simulink model "PMSM_gm_can_outside_Trq_attack"  (R2023a)
settings: Solver=VariableStepAuto  StartTime=0  StopTime=t_sim  RelTol=1e-3
values from neighbouring files (symbols this model uses):
  chosen_cycle = input('Enter the number of the desired driver cycle-choose: \n 1 for Artemis Motorway Driving cycle \n 2 for WHVC \n 3 for ECE urban driving cycle \n 4 for cruise control \n')    [pmsm_g.m]
  J = 0.03    [pmsm_g.m]
  Rated_Cap = 145.5    [pmsm_g.m]
  SOC0 = 1    [pmsm_g.m]
  T_peak = 450    [pmsm_g.m]
  Tire_rad = 0.33435    [pmsm_g.m]
undefined symbols (not defined in the file or in its folder): canChannel, DiscIntNeverNeededParam, sigbuilder_block
libraries: fl_lib x26, nesl_utility x13, sdl_lib x10, canlib x9, canmsglib x8, autolibshared x4, batteryecm_lib x2, ee_lib x2, simulink x1, SignalEditorBlockLib x1
(part 1 of 2)
settings Model: Creator=SMISTOKI  LastModifiedBy=Sadek
settings DebuggingCC: AlgebraicLoopMsg=none

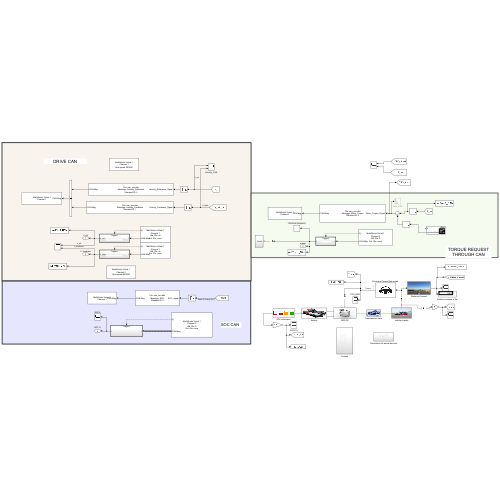
[thumbnail: Simulink's stored preview of the top-level diagram]
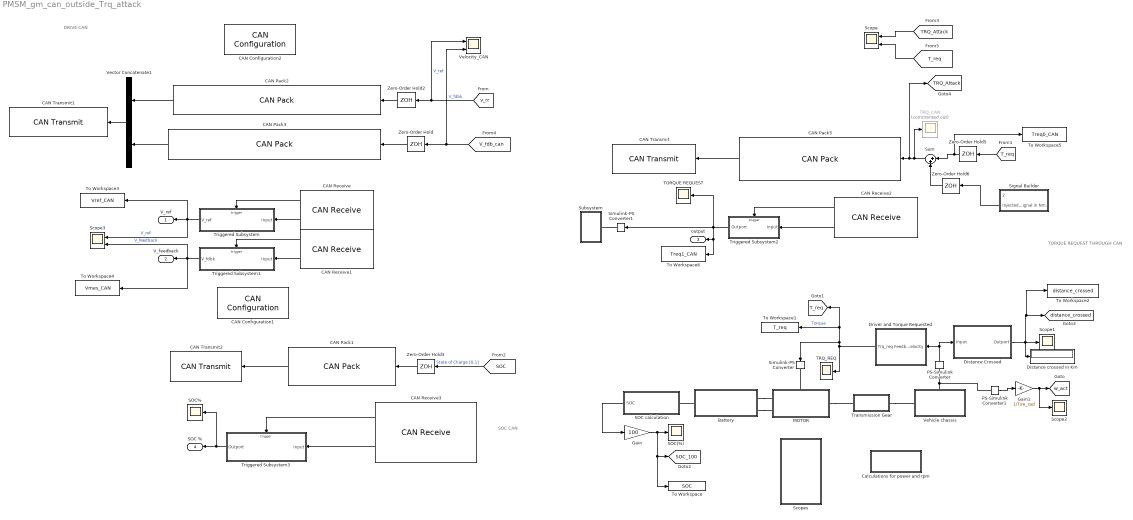
== system PMSM_gm_can_outside_Trq_attack ==
  note: SOC CAN
  note: TORQUE REQUEST THROUGH CAN
  note: DRIVE CAN
  Battery : Subsystem
      settings: PortSchema="{\"entries\":[{\"content\":{\"sides\":[{\"content\":{},\"type\":\"ConnectorPlacement.EquallySpacedRectSide\",\"uuid\":\"d6ab2843-64d8-482c-9d15-215691b6cf54\"},{\"content\":{\"side\":\"RIGHT\"},\"type\":\"ConnectorPlacement.EquallySpacedRectSide\",\"uuid\":\"de85a474-0fdd-49ed-84f8-84d3f4b19d16\"},{\"content\":{\"connectorIds\":[\"LConn1\",\"LConn2\"],\"side\":\"TOP\"},\"type\":\"ConnectorPlacement.EquallySpacedRectSide\",\"uuid\":\"2ee0526d-0566-4e29-bcb7-1bed3def4007\"},{\"content\":{\"connectorIds\":[\"RConn1\"],\"side\":\"BOTTOM\"},\"type\":\"ConnectorPlacement.EquallySpacedRectSide\",\"uuid\":\"606897e6-0cfb-4cd6-a0a0-49c9c925cf1d\"}]},\"type\":\"ConnectorPlacement.EquallySpacedConnector\",\"uuid\":\"bf6b65d6-9bac-4f3f-a275-26fa16d307ff\"}],\"packageUris\":[\"http://schema.mathworks.com/mf0/Connector/R2020b\"],\"version\":\"1.0\"}"
      mask Display: image('$imagefile'); % Use "Edit Image" on toolstrip to change.
  CAN Configuration1 : canlib/CAN Configuration  BlockHandle=30.0001  Device=MathWorks Virtual 1 (Channel 2)  DeviceMenu=MathWorks Virtual 1 (Channel 2)  ObjConstructor=canChannel('MathWorks', 'Virtual 1', 2)  BusSpeed=500000  EnableBitParameters=off  AckMode=Normal
  CAN Configuration2 : canlib/CAN Configuration  BlockHandle=31.0001  Device=MathWorks Virtual 1 (Channel 1)  DeviceMenu=MathWorks Virtual 1 (Channel 1)  ObjConstructor=canChannel('MathWorks', 'Virtual 1', 1)  BusSpeed=500000  EnableBitParameters=off  AckMode=Normal
  CAN Pack1 : canmsglib/CAN Pack  CANdbFile=C:\Users\Sadek\OneDrive - Politecnico di Torino\Final model\can_ecu.dbc  MsgList=SOC  MsgName=SOC  MsgIDType=Standard (11-bit identifier)  MsgIdentifier=5  MsgLength=8  Remote=off  ApplyMinMax=off  BusOutput=off  SignalInfo={'SOC_signal','0','64','LE','double','Standard','0','1','-20','0','100'}
      settings: LibrarySourceBlock=canlib/CAN Pack  DataFormat=CANdb specified signals
  CAN Pack2 : canmsglib/CAN Pack  CANdbFile=C:\Users\Sadek\OneDrive - Politecnico di Torino\Final model\can_ecu.dbc  MsgList=Velocity_Reference  MsgName=Velocity_Reference  MsgIDType=Standard (11-bit identifier)  MsgIdentifier=2  MsgLength=8  Remote=off  ApplyMinMax=off  BusOutput=off  SignalInfo={'Velocity_Reference_Signal','0','64','LE','double','Standard','0','1','-20','0','10000'}
      settings: LibrarySourceBlock=canlib/CAN Pack  DataFormat=CANdb specified signals
  CAN Pack3 : canmsglib/CAN Pack  CANdbFile=C:\Users\Sadek\OneDrive - Politecnico di Torino\Final model\can_ecu.dbc  MsgList=Velocity_Feedback  MsgName=Velocity_Feedback  MsgIDType=Standard (11-bit identifier)  MsgIdentifier=1  MsgLength=8  Remote=off  ApplyMinMax=off  BusOutput=off  SignalInfo={'Velocity_Feedback_Signal','0','64','LE','double','Standard','0','1','-20','0','10000'}
      settings: LibrarySourceBlock=canlib/CAN Pack  DataFormat=CANdb specified signals
  CAN Pack5 : canmsglib/CAN Pack  CANdbFile=C:\Users\Sadek\OneDrive - Politecnico di Torino\Final model\can_ecu.dbc  MsgList=Motor_Torque  MsgName=Motor_Torque  MsgIDType=Standard (11-bit identifier)  MsgIdentifier=0  MsgLength=8  Remote=off  ApplyMinMax=off  BusOutput=off  SignalInfo={'Motor_Torque_Signal','0','64','LE','signed','Standard','0','1','-20','-50000','50000'}
      settings: LibrarySourceBlock=canlib/CAN Pack  DataFormat=CANdb specified signals
  CAN Receive : canlib/CAN Receive  BlockHandle=44.0001  Device=MathWorks Virtual 1 (Channel 1)  DeviceMenu=MathWorks Virtual 1 (Channel 1)  ObjConstructor=canChannel('MathWorks', 'Virtual 1', 1)  EnableStandardIDsFilter=off  StdIDsCombo=Allow all  StandardIDs=0  EnableExtendedIDsFilter=off  ExtIDsCombo=Block all  ExtendedIDs=0  SampleTime=0.01  MsgsPerTimestep=all  InternalFilterUpdateStatus=on  BusOutput=off
  CAN Receive1 : canlib/CAN Receive  BlockHandle=47.0001  Device=MathWorks Virtual 1 (Channel 1)  DeviceMenu=MathWorks Virtual 1 (Channel 1)  ObjConstructor=canChannel('MathWorks', 'Virtual 1', 1)  EnableStandardIDsFilter=off  StdIDsCombo=Allow all  StandardIDs=0  EnableExtendedIDsFilter=off  ExtIDsCombo=Block all  ExtendedIDs=0  SampleTime=0.01  MsgsPerTimestep=all  InternalFilterUpdateStatus=on  BusOutput=off
  CAN Receive2 : canlib/CAN Receive  BlockHandle=50.0001  Device=MathWorks Virtual 1 (Channel 2)  DeviceMenu=MathWorks Virtual 1 (Channel 2)  ObjConstructor=canChannel('MathWorks', 'Virtual 1', 2)  EnableStandardIDsFilter=off  StdIDsCombo=Allow only  StandardIDs=0  EnableExtendedIDsFilter=off  ExtIDsCombo=Block all  ExtendedIDs=0  SampleTime=0.01  MsgsPerTimestep=all  InternalFilterUpdateStatus=on  BusOutput=off
  CAN Receive3 : canlib/CAN Receive  BlockHandle=53.0001  Device=MathWorks Virtual 1 (Channel 2)  DeviceMenu=MathWorks Virtual 1 (Channel 2)  ObjConstructor=canChannel('MathWorks', 'Virtual 1', 2)  EnableStandardIDsFilter=off  StdIDsCombo=Allow only  StandardIDs=5  EnableExtendedIDsFilter=off  ExtIDsCombo=Block all  ExtendedIDs=0  SampleTime=0.01  MsgsPerTimestep=all  InternalFilterUpdateStatus=on  BusOutput=on
  CAN Transmit : canlib/CAN Transmit  BlockHandle=56.0001  Device=MathWorks Virtual 1 (Channel 1)  DeviceMenu=MathWorks Virtual 1 (Channel 1)  ObjConstructor=canChannel('MathWorks', 'Virtual 1', 1)  EnableEventTransmit=off  EnablePeriodicTransmit=off  MessagePeriod=1.000
  CAN Transmit1 : canlib/CAN Transmit  BlockHandle=58.0001  Device=MathWorks Virtual 1 (Channel 1)  DeviceMenu=MathWorks Virtual 1 (Channel 1)  ObjConstructor=canChannel('MathWorks', 'Virtual 1', 1)  EnableEventTransmit=off  EnablePeriodicTransmit=off  MessagePeriod=1.000
  CAN Transmit2 : canlib/CAN Transmit  BlockHandle=60.0001  Device=MathWorks Virtual 1 (Channel 1)  DeviceMenu=MathWorks Virtual 1 (Channel 1)  ObjConstructor=canChannel('MathWorks', 'Virtual 1', 1)  EnableEventTransmit=off  EnablePeriodicTransmit=off  MessagePeriod=1.000
  Calculations for power and rpm : Subsystem
  Distance Crossed : Subsystem
      mask Display: image('$imagefile'); % Use "Edit Image" on toolstrip to change.
  Distance crossed in Km : Display
  "Driver and Torque Requested " : Subsystem
      mask Display: image('$imagefile'); % Use "Edit Image" on toolstrip to change.
  Gain : Gain  Gain=100
  Gain1 : Gain  Gain=1/Tire_rad
  MOTOR : Subsystem
      settings: PortSchema="{\"entries\":[{\"content\":{\"sides\":[{\"content\":{\"connectorIds\":[\"LConn1\",\"LConn2\"]},\"type\":\"ConnectorPlacement.EquallySpacedRectSide\",\"uuid\":\"2895f6cb-f09c-4811-a438-7c51f6a6223f\"},{\"content\":{\"connectorIds\":[\"RConn1\"],\"side\":\"RIGHT\"},\"type\":\"ConnectorPlacement.EquallySpacedRectSide\",\"uuid\":\"62dfe04d-e035-47c8-a996-d867f35d8ae8\"},{\"content\":{\"connectorIds\":[\"LConn3\"],\"side\":\"TOP\"},\"type\":\"ConnectorPlacement.EquallySpacedRectSide\",\"uuid\":\"0c3302b4-833a-415e-90fd-2f2c79a3935c\"}]},\"type\":\"ConnectorPlacement.EquallySpacedConnector\",\"uuid\":\"ac0404f8-73ea-47f6-91f8-dc1d39a3ba60\"}],\"packageUris\":[\"http://schema.mathworks.com/mf0/Connector/R2020b\"],\"version\":\"1.0\"}"
      mask Display: image('$imagefile'); % Use "Edit Image" on toolstrip to change.
  PS-Simulink Converter : nesl_utility/PS-Simulink Converter  PhysicalDomain=network_engine_domain  SubClassName=ps_output  LeftPortType=input  RightPortType=output  PseudoPeriodic=off  Frequencies=[]  VectorFormat=inherit  Unit=inherit  AffineConversion=off
  PS-Simulink Converter1 : nesl_utility/PS-Simulink Converter  PhysicalDomain=network_engine_domain  SubClassName=ps_output  LeftPortType=input  RightPortType=output  PseudoPeriodic=off  Frequencies=[]  VectorFormat=inherit  Unit=inherit  AffineConversion=off
  "SOC calculation " : Subsystem
      mask Display: image('$imagefile'); % Use "Edit Image" on toolstrip to change.
  SOC% : Scope
  SOC(%) : Scope
  Scope : Scope  NumInputPorts=2
  Scope1 : Scope
  Scope2 : Scope
  Scope3 : Scope  NumInputPorts=2
  Scopes : Subsystem
  Signal Builder : Subsystem  Tag=STV Subsys  LoadFcn=sigbuilder_block('load');  StartFcn=sigbuilder_block('start');  StopFcn=sigbuilder_block('stop');  ClipboardFcn=sigbuilder_block('clipboard');  mask(Sigbuilder block){tuvar=[0:10]}
      mask help: Simulink:masks:SigbuilderBlock_MD
      mask init:
      | if ~strcmp(get_param(bdroot(gcbh),'SimulationStatus'),'stopped') tuvar = sigbuilder_block('maskInit'); end
      settings: CopyFcn=sigbuilder_block('copy');  DeleteFcn=sigbuilder_block('delete');  ModelCloseFcn=sigbuilder_block('modelClose');  PreSaveFcn=sigbuilder_block('preSave');  PauseFcn=sigbuilder_block('pause');  ContinueFcn=sigbuilder_block('continue');  NameChangeFcn=sigbuilder_block('namechange');  OpenFcn=sigbuilder_block('open',[5.4 5.4 1141.2 580.8 ]);  CloseFcn=sigbuilder_block('close');
      mask Display: plot(0, 0, 100, 100,[2, 2, 32, 32, 2], [68, 8, 8, 68, 68],[32, 2], [38, 38], [32, 19, 2],[53, 60, 44], [32, 17, 17, 2],[16, 16, 31, 31]);txt = getActiveGroup(gcbh);text(2, 100, txt,'verticalAlignment', 'top');
  Simulink-PS Converter : nesl_utility/Simulink-PS Converter  PhysicalDomain=network_engine_domain  SubClassName=ps_input  LeftPortType=input  RightPortType=output  PseudoPeriodic=off  Frequencies=[]  NoiseDistribution=none  NoiseParameters=[]  Unit=1  AffineConversion=off  FilteringAndDerivatives=provide  SimscapeFilterOrder=1  InputFilterTimeConstant=0.001  UdotUserProvided=0
  Simulink-PS Converter1 : nesl_utility/Simulink-PS Converter  PhysicalDomain=network_engine_domain  SubClassName=ps_input  LeftPortType=input  RightPortType=output  PseudoPeriodic=off  Frequencies=[]  NoiseDistribution=none  NoiseParameters=[]  Unit=1  AffineConversion=off  FilteringAndDerivatives=provide  SimscapeFilterOrder=1  InputFilterTimeConstant=0.001  UdotUserProvided=0
  Subsystem : Subsystem
  Sum : Sum  Inputs=|++
  TORQUE REQUEST : Scope
  TRQ_CAN : Scope  Commented=on
  TRQ_REQ : Scope
  To Workspace : ToWorkspace  VariableName=SOC  SaveFormat=Timeseries  SampleTime=-1
  To Workspace1 : ToWorkspace  VariableName=T_req  SaveFormat=Timeseries  SampleTime=-1
  To Workspace2 : ToWorkspace  VariableName=distance_crossed  SaveFormat=Timeseries  SampleTime=-1
  To Workspace3 : ToWorkspace  VariableName=Vref_CAN  SaveFormat=Timeseries  SampleTime=-1
  To Workspace4 : ToWorkspace  VariableName=Vmes_CAN  SaveFormat=Timeseries  SampleTime=-1
  To Workspace5 : ToWorkspace  VariableName=Treq0_CAN  SaveFormat=Timeseries  SampleTime=-1
  To Workspace6 : ToWorkspace  VariableName=Treq1_CAN  SaveFormat=Timeseries  SampleTime=-1
  Transmission Gear : Subsystem
      mask Display: image('$imagefile'); % Use "Edit Image" on toolstrip to change.
  Triggered Subsystem : Subsystem  TreatAsAtomicUnit=on
      settings: LibrarySourceBlock=|
      | hdlsllib/Ports &
      | Subsystems/Triggered
      | Subsystem
  Triggered Subsystem1 : Subsystem  TreatAsAtomicUnit=on
      settings: LibrarySourceBlock=|
      | hdlsllib/Ports &
      | Subsystems/Triggered
      | Subsystem
  Triggered Subsystem2 : Subsystem  TreatAsAtomicUnit=on
      settings: LibrarySourceBlock=|
      | hdlsllib/Ports &
      | Subsystems/Triggered
      | Subsystem
  Triggered Subsystem3 : Subsystem  TreatAsAtomicUnit=on
  Vector Concatenate1 : Concatenate
  Vehicle chassis : Subsystem
      settings: PortSchema="{\"entries\":[{\"content\":{\"sides\":[{\"content\":{\"connectorIds\":[\"LConn1\"]},\"type\":\"ConnectorPlacement.EquallySpacedRectSide\",\"uuid\":\"cbb2d22d-924c-423d-830f-e93cab1699a7\"},{\"content\":{\"side\":\"RIGHT\"},\"type\":\"ConnectorPlacement.EquallySpacedRectSide\",\"uuid\":\"50d26a31-cf69-4945-8446-5696a2ab25a5\"},{\"content\":{\"connectorIds\":[\"LConn2\"],\"side\":\"TOP\"},\"type\":\"ConnectorPlacement.EquallySpacedRectSide\",\"uuid\":\"4303cca7-e79c-4b33-9500-6ba7c742b47b\"}]},\"type\":\"ConnectorPlacement.EquallySpacedConnector\",\"uuid\":\"a196d690-580d-41dc-a9f1-902992004778\"}],\"packageUris\":[\"http://schema.mathworks.com/mf0/Connector/R2020b\"],\"version\":\"1.0\"}"
      mask Display: image('$imagefile'); % Use "Edit Image" on toolstrip to change.
  Velocity_CAN : Scope  NumInputPorts=2
  Zero-Order Hold{,2..3,5..6} (5 alike) : ZeroOrderHold  SampleTime=0.1
  V_ref : Outport
  V_feedback : Outport  Port=2
  output : Outport  Port=3
  SOC % : Outport  Port=4
  tag scope: SOC_100=global, TRQ_Attack=global, T_req=global, distance_crossed=global, w_act=global
  wires:
  PS-Simulink Converter/1 -> Distance Crossed/1(Input), "Driver and Torque Requested "/1(Feedback Velocity)
  "SOC calculation "/1(SOC) -> Gain/1
  Gain/1 -> To Workspace/1, [SOC_100], SOC(%)/1
  Distance Crossed/1(Outport) -> To Workspace2/1, [distance_crossed], Scope1/1, Distance crossed in Km/1
  "Driver and Torque Requested "/1(Trq_req) -> To Workspace1/1, [T_req], Simulink-PS Converter/1, TRQ_REQ/1  "Torque"
  PS-Simulink Converter1/1 -> Gain1/1
  Gain1/1 -> Scope2/1, [w_act]
  [v_rr] -> Velocity_CAN/1, Zero-Order Hold2/1  "V_ref"
  CAN Receive/1 -> Triggered Subsystem/Trigger
  CAN Receive/2 -> Triggered Subsystem/1(Input)
  CAN Receive1/2 -> Triggered Subsystem1/1(Input)
  CAN Receive1/1 -> Triggered Subsystem1/Trigger
  Triggered Subsystem1/1(V_fdbk) -> To Workspace4/1, Scope3/2, V_feedback/1  "V_feedback"
  Triggered Subsystem/1(V_ref) -> To Workspace3/1, Scope3/1, V_ref/1  "V_ref"
  CAN Pack3/1 -> Vector Concatenate1/2
  Zero-Order Hold/1 -> CAN Pack3/1
  Vector Concatenate1/1 -> CAN Transmit1/1
  CAN Pack2/1 -> Vector Concatenate1/1
  Zero-Order Hold2/1 -> CAN Pack2/1
  CAN Receive2/1 -> Triggered Subsystem2/Trigger
  CAN Receive2/2 -> Triggered Subsystem2/1(Input)
  CAN Pack1/1 -> CAN Transmit2/1
  [SOC] -> Zero-Order Hold3/1  "State of Charge [0,1]"
  CAN Receive3/1 -> Triggered Subsystem3/Trigger
  CAN Receive3/2 -> Triggered Subsystem3/1(Input)
  Triggered Subsystem3/1(Outport) -> SOC%/1, SOC %/1
  Zero-Order Hold3/1 -> CAN Pack1/1
  CAN Pack5/1 -> CAN Transmit/1
  [T_req] -> Zero-Order Hold5/1
  Zero-Order Hold6/1 -> Sum/2
  Sum/1 -> TRQ_CAN/1, [TRQ_Attack], CAN Pack5/1
  [V_fdb_can] -> Velocity_CAN/2, Zero-Order Hold/1  "V_fdbk"
  Zero-Order Hold5/1 -> To Workspace5/1, Sum/1
  Triggered Subsystem2/1(Outport) -> To Workspace6/1, output/1, TORQUE REQUEST/1, Simulink-PS Converter1/1
  Signal Builder/2(Injected Attacking Signal in Nm.) -> Zero-Order Hold6/1
  [TRQ_Attack] -> Scope/1
  [T_req] -> Scope/2
  connections:
  Transmission Gear/RConn1 -- Vehicle chassis/LConn1
  MOTOR/LConn3 -- Simulink-PS Converter/RConn1
  PS-Simulink Converter/LConn1 -- PS-Simulink Converter1/LConn1 -- Vehicle chassis/LConn2
  Battery/RConn1 -- "SOC calculation "/LConn1
  Battery/LConn1 -- MOTOR/LConn1
  Battery/LConn2 -- MOTOR/LConn2
  MOTOR/RConn1 -- Transmission Gear/LConn1
  Simulink-PS Converter1/RConn1 -- Subsystem/LConn1

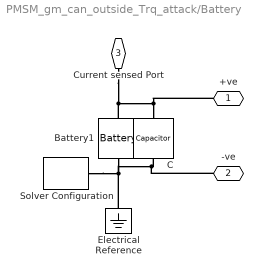
== system PMSM_gm_can_outside_Trq_attack/Battery ==
  Battery1 : batteryecm_lib/Battery  Vnom=Vnom V  prm_dir=simscape.enum.battery.prm_dir.disabled  R1_dis=2 Ohm  R1_ch=2 Ohm  R1=R_internal Ohm  prm_AH=simscape.enum.battery.prm_AH.finite  AH=Rated_Cap A*hr  V1=V1 V  AH1=AH1 A*hr  prm_R2=simscape.enum.battery.prm_R2.enabled  R2=2000 Ohm  Tmeas=298.15 K  charge_measurement_port=simscape.enum.battery.enable.no  prm_dyn=simscape.enum.battery.prm_dyn.off  Rp1=0.005 Ohm  tau1=30 s  Rp2=0.005 Ohm  tau2=30 s  Rp3=0.005 Ohm  tau3=30 s  Rp4=0.005 Ohm  tau4=30 s  Rp5=0.005 Ohm  tau5=30 s  prm_fade=simscape.enum.battery.prm_fade.disabled  N_fade=100  AH_fade=45 A*hr  R1_fade=2.02 Ohm  R1_ch_fade=2.02 Ohm  V1_fade=10.35 V  prm_age=simscape.enum.battery.prm_age.disabled  prm_age_OCV=simscape.enum.battery.prm_age_OCV.OCV  OCV_age=0.9  SOC_age=60  Tmeas_age=298.15 K  delta_time_age_vec=[0] d  temperature_age_vec=[273] K  OCV_scaling_age=2.2134e6  OCV_offset_age=1.632e6  temp_exp_age=0.515833569 V  t_exp_age=0.75  Vnom_T2=12 V  R1_T2=2.2 Ohm  R1_T2_dis=2.2 Ohm  R1_T2_ch=2.2 Ohm  V1_T2=11.4 V  R2_T2=2200 Ohm  Rp1_T2=0.005 Ohm  tau1_T2=30 s  Rp2_T2=0.005 Ohm  tau2_T2=30 s  Rp3_T2=0.005 Ohm  tau3_T2=30 s  Rp4_T2=0.005 Ohm  tau4_T2=30 s  Rp5_T2=0.005 Ohm  tau5_T2=30 s  Tmeas2=273.15 K  thermal_port=simscape.enum.thermaleffects.omit  thermal_mass=30000 J/K  i_specify=off  i_priority=None  i=0 A  i_nominal_specify=off  i_nominal_unit=A  i_nominal_value=1  v_specify=off  v_priority=None  v=0 V  v_nominal_specify=off  v_nominal_unit=V  v_nominal_value=1  charge_specify=off  charge_priority=High  charge=50 A*hr  charge_nominal_specify=off  charge_nominal_unit=A*hr  charge_nominal_value=1  num_cycles_specify=off  num_cycles_priority=High  num_cycles=0  num_cycles_nominal_specify=off  num_cycles_nominal_unit=1  num_cycles_nominal_value=1  temperature_specify=off  temperature_priority=High  temperature=298.15 K  temperature_nominal_specify=off  temperature_nominal_unit=K  temperature_nominal_value=1
  C : fl_lib/Electrical/Electrical Elements/Capacitor  c=Cdc F  r=1e-6 Ohm  g=0 1/Ohm  i_specify=off  i_priority=None  i=0 A  i_nominal_specify=off  i_nominal_unit=A  i_nominal_value=1  v_specify=off  v_priority=None  v=0 V  v_nominal_specify=on  v_nominal_unit=V  v_nominal_value=Vcdc0  vc_specify=on  vc_priority=High  vc=Vcdc0 V  vc_nominal_specify=off  vc_nominal_unit=V  vc_nominal_value=1
  Electrical Reference : fl_lib/Electrical/Electrical Elements/Electrical Reference
  Solver Configuration : nesl_utility/Solver Configuration  PhysicalDomain=network_engine_domain  SubClassName=solver  LeftPortType=input  RightPortType=generic  Tones=[]  Harmonics=[]  SimulateNoise=off  Profile=off  UseLocalSampling=off  EnableSwitchedLinearOptims=on  FrequencyDomain=off  UseCCode=off  RelTol=0.001  AbsTol=0.001  MinStep=1e-09  ToWorkspace=off  RevertToSquareIcSolve=off  NumHomotopyIterations=100  PhasorMode=off  PhasorModeNumHarmonics=1  ConsistencySolver=NEWTON_XTOL_AFTER_FTOL  IndexReductionMethod=DerivativeReplacement  DoDC=off  ResidualTolerance=1e-09  ConsistencyTolSource=GLOBAL  ConsistencyAbsTol=0.001  ConsistencyRelTol=0.001  ConsistencyTolFactor=0.001  UseLocalSolver=off  LocalSolverChoice=NE_BACKWARD_EULER_ADVANCER  ResolveIndetEquations=on  FunctionEvalNumThread=1  LocalSolverSampleTime=0.001  DoFixedCost=off  MaxNonlinIter=3  MaxModeIter=2  ComputeImpulses=off  ImpulseIterations=2  LinearAlgebra=auto  LinearAlgebraNumThread=0  EquationFormulation=NE_TIME_EF  DelaysMemoryBudget=1024  AutomaticFiltering=on  FilteringTimeConstant=0.001  PartitionStorageMethod=AS_NEEDED  PartitionMemoryBudget=1024  PartitionMethod=ROBUST
  +ve : PMIOPort  Side=Left
  -ve : PMIOPort  Port=2  Side=Left
  Current sensed Port : PMIOPort  Port=3  Side=Right
  connections:
  Electrical Reference/LConn1 -- Solver Configuration/RConn1 -- -ve/RConn1 -- C/RConn1 -- Battery1/RConn1
  Battery1/LConn1 -- +ve/RConn1 -- C/LConn1 -- Current sensed Port/RConn1

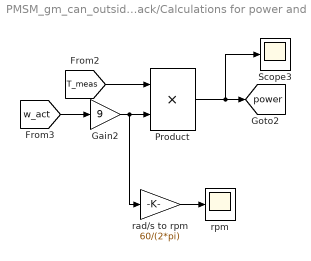
== system PMSM_gm_can_outside_Trq_attack/Calculations for power and rpm ==
  Gain2 : Gain  Gain=9
  Product : Product
  Scope3 : Scope
  rad/s to rpm : Gain  Gain=60/(2*pi)
  rpm : Scope
  tag scope: power=global
  wires:
  Product/1 -> Scope3/1, [power]
  rad/s to rpm/1 -> rpm/1
  [w_act] -> Gain2/1
  [T_meas] -> Product/1
  Gain2/1 -> rad/s to rpm/1, Product/2

== system PMSM_gm_can_outside_Trq_attack/Distance Crossed ==
  Input : Inport
  Integrator : Integrator
  m->km : Gain  Gain=1e-3
  Outport : Outport
  wires:
  Integrator/1 -> m->km/1
  m->km/1 -> Outport/1
  Input/1 -> Integrator/1

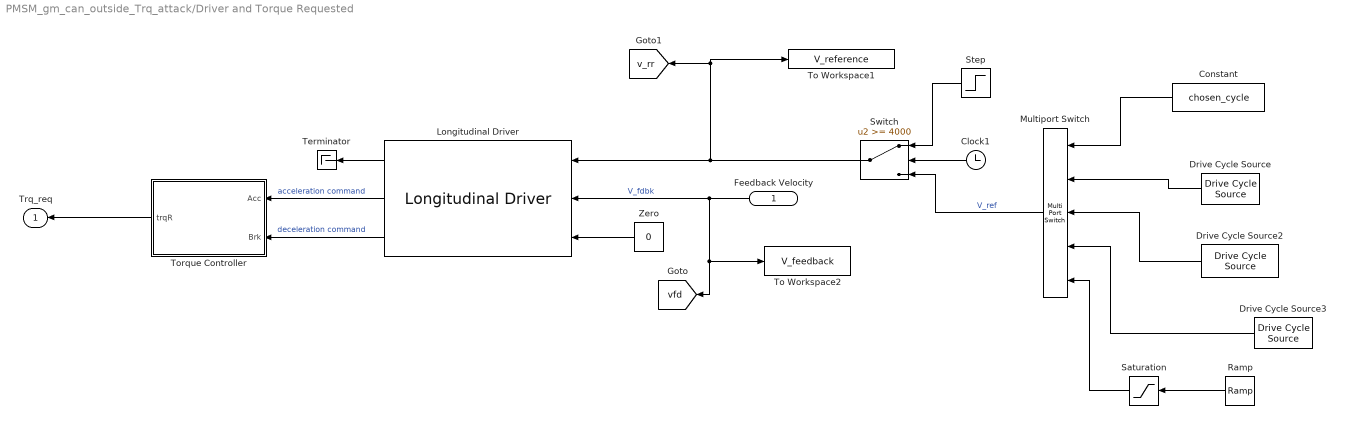
== system PMSM_gm_can_outside_Trq_attack/Driver and Torque Requested  ==
  Feedback Velocity : Inport
  Clock1 : Clock
  Constant : Constant  Value=chosen_cycle
  Drive Cycle Source : autolibshared/Drive Cycle Source  cycleVar=Artemis Motorway 130 kmph  fileVar=cycleFTP75.mat  tfinal="1068  seconds"  cycleRepeat=off  outAccPort=off  outGearPort=off  gearList=No gear data  t_wot1=5  xdot_woto=0  xdot_wot1=30  t_wot2=20  xdot_wot2=0  t_wotend=30  srcUnit=m/s  outUnit=m/s  srcAccUnit=m/s/s  outAccUnit=m/s^2  dt=0  aMode=1  faultOption=off  velBnd=2  velBndUnit=mph  inUnit=m/s  timeBnd=1  failOption=off  stopSim=off  maxFaultCnt=10  maxFaultTime=2  maxTotFaultTime=15  traceOption=off  dtTrace=1  traceWindow=10  lastDCname=Artemis Motorway 130 kmph  lastOutUnit=mph  lastDT=0  lastTB=1  lastSB=2  forceCalcBound=off
  Drive Cycle Source2 : autolibshared/Drive Cycle Source  cycleVar=World Harmonized Vehicle Cycle (WHVC)  fileVar=cycleFTP75.mat  tfinal="900  seconds"  cycleRepeat=off  outAccPort=off  outGearPort=off  gearList=No gear data  t_wot1=5  xdot_woto=0  xdot_wot1=30  t_wot2=20  xdot_wot2=0  t_wotend=30  srcUnit=m/s  outUnit=m/s  srcAccUnit=m/s/s  outAccUnit=m/s^2  dt=0  aMode=1  faultOption=off  velBnd=2  velBndUnit=mph  inUnit=m/s  timeBnd=1  failOption=off  stopSim=off  maxFaultCnt=10  maxFaultTime=2  maxTotFaultTime=15  traceOption=off  dtTrace=1  traceWindow=10  lastDCname=World Harmonized Vehicle Cycle (WHVC)  lastOutUnit=mph  lastDT=0  lastTB=1  lastSB=2  forceCalcBound=off
  Drive Cycle Source3 : autolibshared/Drive Cycle Source  cycleVar=ECE Extra-Urban Driving Cycle (Low Powered Vehicles)  fileVar=cycleFTP75.mat  tfinal="400  seconds"  cycleRepeat=off  outAccPort=off  outGearPort=off  gearList=No gear data  t_wot1=5  xdot_woto=0  xdot_wot1=30  t_wot2=20  xdot_wot2=0  t_wotend=30  srcUnit=m/s  outUnit=m/s  srcAccUnit=m/s/s  outAccUnit=m/s^2  dt=0  aMode=1  faultOption=off  velBnd=2  velBndUnit=mph  inUnit=m/s  timeBnd=1  failOption=off  stopSim=off  maxFaultCnt=10  maxFaultTime=2  maxTotFaultTime=15  traceOption=off  dtTrace=1  traceWindow=10  lastDCname=ECE Extra-Urban Driving Cycle (Low Powered Vehicles)  lastOutUnit=mph  lastDT=0  lastTB=1  lastSB=2  forceCalcBound=off
  Longitudinal Driver : autolibshared/Longitudinal Driver  extAccelOvr=off  extDecelOvr=off  extAccelHld=off  extDecelHld=off  extAccelZero=off  extDecelZero=off  cntrlType=PI  shftType=None  velUnits=m/s  gearOut=off  Kp=100  Ki=30  Kff=.05  Kg=.01  VehVelVec=[0 100]  KffVec=[.1 .1]  KpVec=[10 10]  KiVec=[5 5]  KgVec=[0 0]  m=1500  Kpt=3000  tau=.1  L=2  aR=200  bR=2.5  cR=.5  g=9.81  vnom=100  Kaw=.1  tauerr=.03  tauPt=2  GearInit=0  tShift=.1  pdlVec=[0.1 0.4 0.5 0.9]  upShftTbl=[-1 12.9375 26.4375 39.9375 51.18749999999999 62.4375 72.84375 83.25;-1 16.3125 29.8125 43.3125 54.5624 65.8125 76.78125 87.75;-1 19.6875 33.1875 46.68749999999999 57.9375 69.1875 80.71875 92.25;-1 33 52.5 77.25 100.5 138.75 161.875 185]  dwnShftTbl=[1 9.5625 23.0625 36.5625 47.8125 59.0625 68.90625 78.75;1 12.9375 26.4375 39.9375 51.18749999999999 62.4375 72.84375 83.25;1 16.3125 29.8125 43.3125 54.562499 65.8125 76.78125 87.75;1 19.6875 33.1875 46.68749999999999 57.9375 69.1875 80.71875 92.25]  tClutch=.5  tRev=.5  tPark=120  aMode=1  UpGearVec="[0  1  2  3  4  5  6  7]"  DownGearVec="[1  2  3  4  5  6  7  8]"
  Multiport Switch : MultiPortSwitch  Inputs=4  SaturateOnIntegerOverflow=off  InputSameDT=off
  Ramp : simulink/Sources/Ramp  slope=1  start=0  InitialOutput=0
  Saturation : Saturate  UpperLimit=28  LowerLimit=0
  Step : Step  Time=100  Before=10  After=20  SampleTime=0
  Switch : Switch  Threshold=4000  SaturateOnIntegerOverflow=off  InputSameDT=off
  Terminator : Terminator
  To Workspace1 : ToWorkspace  VariableName=V_reference  SaveFormat=Timeseries  SampleTime=-1
  To Workspace2 : ToWorkspace  VariableName=V_feedback  SaveFormat=Timeseries  SampleTime=-1
  Torque Controller : Subsystem
  Zero : Constant  Value=0  OutDataTypeStr=Inherit: Inherit via back propagation
  Trq_req : Outport
  tag scope: v_rr=global, vfd=global
  wires:
  Longitudinal Driver/1 -> Terminator/1
  Longitudinal Driver/2 -> Torque Controller/1(Acc)  "acceleration command"
  Longitudinal Driver/3 -> Torque Controller/2(Brk)  "deceleration command"
  Torque Controller/1(trqR) -> Trq_req/1
  Zero/1 -> Longitudinal Driver/3
  Feedback Velocity/1 -> Longitudinal Driver/2, To Workspace2/1, [vfd]  "V_fdbk"
  Clock1/1 -> Switch/2
  Multiport Switch/1 -> Switch/3  "V_ref"
  Step/1 -> Switch/1
  Switch/1 -> [v_rr], To Workspace1/1, Longitudinal Driver/1
  Drive Cycle Source2/1 -> Multiport Switch/3
  Drive Cycle Source3/1 -> Multiport Switch/4
  Drive Cycle Source/1 -> Multiport Switch/2
  Constant/1 -> Multiport Switch/1
  Ramp/1 -> Saturation/1
  Saturation/1 -> Multiport Switch/5

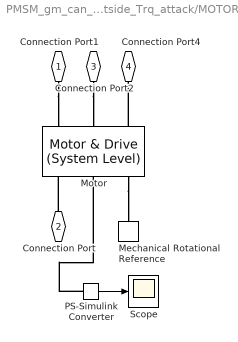
== system PMSM_gm_can_outside_Trq_attack/MOTOR ==
  Mechanical Rotational Reference : fl_lib/Mechanical/Rotational Elements/Mechanical Rotational Reference
  Motor : ee_lib/Electromechanical/Motor & Drive (System Level)  torque_speed_param=ee.enum.electromech.envelope.torque_power  overtorque_param=ee.enum.electromech.overtorque.no  T_t=[.09, .08, .07, 0] N*m  T_t_intermittent=[.36, .32, .28, 0] N*m  T_t_2D=[.09, .09, .09; .08, .08, .08; .07, .07, .07; 0, 0, 0] N*m  T_t_intermittent_2D=[.36, .36, .36; .32, .32, .32; .28, .28, .28; 0, 0, 0] N*m  w_t=[0, 3750, 7500, 8000] rpm  vdc_t=[6, 12, 24] V  torque_max=T_peak N*m  power_max=P_peak kW  torque_max_intermittent=0.4 N*m  power_max_intermittent=120 W  time_overtorque=30 s  time_recover=60 s  Tc=Tc s  losses_param=1  eff=efficiency  w_eff=w_eff rpm  T_eff=T_eff N*m  Piron=0 W  Pbase=0 W  w_eff_vec=[-8000, -4000, 0, 4000, 8000] rpm  T_eff_vec=[0, .03, .06, .09] N*m  v_eff_vec=[100, 250, 400] V  losses_mat=[1.49, 1.67, 2.21, 3.1; .42, .69, 1.14, 2.03; .06, .24, .78, 1.68; .42, .69, 1.14, 2.03; 1.49, 1.67, 2.21, 3.1] W  efficiency_mat=[95, 95, 95, 95; 95, 95, 95, 95; 95, 95, 95, 95; 95, 95, 95, 95; 95, 95, 95, 95]  losses_mat_3D=ones(5, 4, 3) W  efficiency_mat_3D=95 * ones(5, 4, 3)  Res=Resistance Ohm  enable_fault=simscape.enum.onoff.off  fault_condition=1  fault_threshold=0.5  J=J kg*m^2  lam=R_damp N*m/(rad/s)  speed0=0 rpm  faulted_specify=off  faulted_priority=None  faulted=0  faulted_nominal_specify=off  faulted_nominal_unit=1  faulted_nominal_value=1  torqueLimitContinuous_specify=off  torqueLimitContinuous_priority=None  torqueLimitContinuous=0 N*m  torqueLimitContinuous_nominal_specify=off  torqueLimitContinuous_nominal_unit=N*m  torqueLimitContinuous_nominal_value=1  alpha=3.93e-3 1/K  Tmeas=25 degC  Tmeas2=125 degC  losses_mat_T2=[1.49, 1.74, 2.49, 3.74; .42, .67, 1.42, 2.67; .06, .31, 1.06, 2.31; .42, .67, 1.42, 2.67; 1.49, 1.74, 2.49, 3.74] W  efficiency_mat_T2=[95, 95, 95, 95; 95, 95, 95, 95; 95, 95, 95, 95; 95, 95, 95, 95; 95, 95, 95, 95]  losses_mat_3D_T2=ones(5, 4, 3) W  efficiency_mat_3D_T2=95 * ones(5, 4, 3)  thermal_mass=100 J/K  initial_temperature=25 degC
  PS-Simulink Converter : nesl_utility/PS-Simulink Converter  PhysicalDomain=network_engine_domain  SubClassName=ps_output  LeftPortType=input  RightPortType=output  PseudoPeriodic=off  Frequencies=[]  VectorFormat=inherit  Unit=inherit  AffineConversion=off
  Scope : Scope
  Connection Port1 : PMIOPort  Side=Left
  Connection Port : PMIOPort  Port=2  Side=Left
  Connection Port2 : PMIOPort  Port=3  Side=Left
  Connection Port4 : PMIOPort  Port=4  Side=Right
  wires:
  PS-Simulink Converter/1 -> Scope/1
  connections:
  Connection Port/RConn1 -- Motor/RConn1
  Connection Port1/RConn1 -- Motor/LConn1
  Connection Port2/RConn1 -- Motor/LConn2
  Motor/LConn3 -- Connection Port4/RConn1
  Motor/RConn3 -- Mechanical Rotational Reference/LConn1
  PS-Simulink Converter/LConn1 -- Motor/RConn2

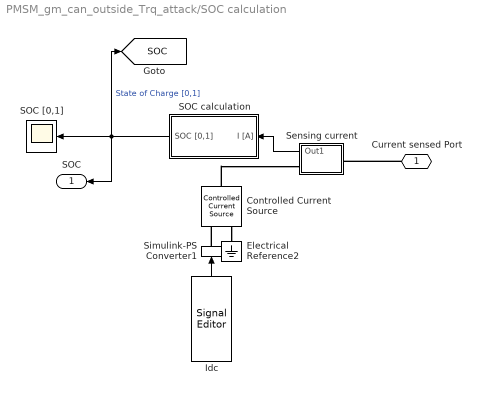
== system PMSM_gm_can_outside_Trq_attack/SOC calculation  ==
  Controlled Current Source : fl_lib/Electrical/Electrical Sources/Controlled Current Source
  Electrical Reference2 : fl_lib/Electrical/Electrical Elements/Electrical Reference
  Idc : SignalEditorBlockLib/Signal Editor  FileName=ee_hv_battery_charge_discharge_Idc.mat  ActiveScenario=Group_1  ActiveSignal=Idc [A]  IsBus=off  OutputBusObjectStr=Bus: BusObject  SampleTime=0  OutputAfterFinalValue=Extrapolation  Unit=inherit  PreserveSignalName=on  ApplySigPropsToAllScenarios=on
  SOC [0,1] : Scope
  SOC calculation : Subsystem
  Sensing current : Subsystem
      mask Display: disp('i')
  Simulink-PS Converter1 : nesl_utility/Simulink-PS Converter  PhysicalDomain=network_engine_domain  SubClassName=ps_input  LeftPortType=input  RightPortType=output  PseudoPeriodic=off  Frequencies=[]  NoiseDistribution=none  NoiseParameters=[]  Unit=A  AffineConversion=off  FilteringAndDerivatives=zero  SimscapeFilterOrder=1  InputFilterTimeConstant=0.001  UdotUserProvided=1
  Current sensed Port : PMIOPort  Side=Left
  SOC : Outport
  tag scope: SOC=global
  wires:
  SOC calculation/1(SOC [0,1]) -> [SOC], SOC/1, SOC [0,1]/1  "State of Charge [0,1]"
  Idc/1 -> Simulink-PS Converter1/1
  Sensing current/1(Out1) -> SOC calculation/1(I [A])
  connections:
  Controlled Current Source/LConn1 -- Sensing current/RConn1
  Simulink-PS Converter1/RConn1 -- Controlled Current Source/RConn1
  Controlled Current Source/RConn2 -- Electrical Reference2/LConn1
  Current sensed Port/RConn1 -- Sensing current/LConn1

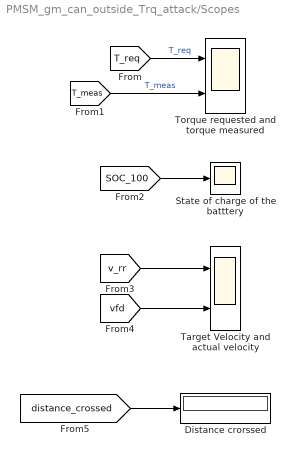
== system PMSM_gm_can_outside_Trq_attack/Scopes ==
  Distance crorssed : Display
  State of charge of the batttery : Scope
  "Target Velocity and actual velocity " : Scope  NumInputPorts=2
  Torque requested and torque measured : Scope  NumInputPorts=2
  wires:
  [T_meas] -> Torque requested and torque measured/2  "T_meas"
  [T_req] -> Torque requested and torque measured/1  "T_req"
  [SOC_100] -> State of charge of the batttery/1
  [v_rr] -> "Target Velocity and actual velocity "/1
  [vfd] -> "Target Velocity and actual velocity "/2
  [distance_crossed] -> Distance crorssed/1

== system PMSM_gm_can_outside_Trq_attack/Signal Builder ==
  Demux : Demux  Tag=STV Demux  Outputs=2
      settings: DisplayOption=none
  FromWs : FromWorkspace  Tag=STV FromWs  VariableName=tuvar
      SigBuilderData=|
      | common.afterFinalStr = 'Extrapolate'
      | common.sampleTime = 0
      | dataSet.timeRange = [0 400]
      | dataSet.name = 'offset'
      | sbobj.Groups.Name = 'offset'
      | sbobj.Groups.Signals(1).Name = '2'
      | sbobj.Groups.Signals(1).XData = [0 40 80 120 150 170 400]
      | sbobj.Groups.Signals(1).YData = [0 136 -70 0 150 -100 0]
      | sbobj.Groups.Signals(2).Name = 'Injected Attacking Signal in Nm.'
      | sbobj.Groups.Signals(2).XData = [0 160 160 240 240 400]
      | sbobj.Groups.Signals(2).YData = [0 0 -15 -15 0 0]
      | sbobj.Groups.TimeRange = [0 400]
  2 : Outport  Tag=STV Outport
  Injected Attacking Signal in Nm. : Outport  Tag=STV Outport  Port=2
  wires:
  FromWs/1 -> Demux/1
  Demux/1 -> 2/1
  Demux/2 -> Injected Attacking Signal in Nm./1

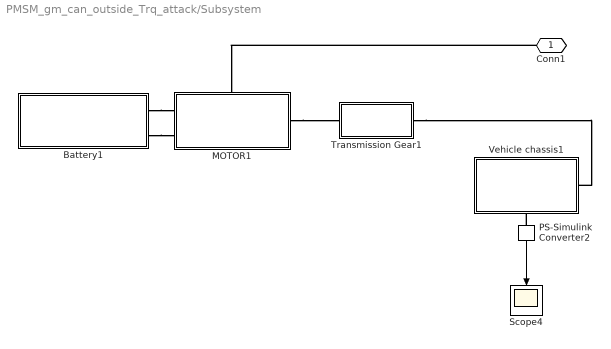
== system PMSM_gm_can_outside_Trq_attack/Subsystem ==
  Battery1 : Subsystem
      settings: PortSchema="{\"entries\":[{\"content\":{\"sides\":[{\"content\":{},\"type\":\"ConnectorPlacement.EquallySpacedRectSide\",\"uuid\":\"d6ab2843-64d8-482c-9d15-215691b6cf54\"},{\"content\":{\"side\":\"RIGHT\"},\"type\":\"ConnectorPlacement.EquallySpacedRectSide\",\"uuid\":\"de85a474-0fdd-49ed-84f8-84d3f4b19d16\"},{\"content\":{\"connectorIds\":[\"LConn1\",\"LConn2\"],\"side\":\"TOP\"},\"type\":\"ConnectorPlacement.EquallySpacedRectSide\",\"uuid\":\"2ee0526d-0566-4e29-bcb7-1bed3def4007\"},{\"content\":{\"side\":\"BOTTOM\"},\"type\":\"ConnectorPlacement.EquallySpacedRectSide\",\"uuid\":\"606897e6-0cfb-4cd6-a0a0-49c9c925cf1d\"}]},\"type\":\"ConnectorPlacement.EquallySpacedConnector\",\"uuid\":\"bf6b65d6-9bac-4f3f-a275-26fa16d307ff\"}],\"packageUris\":[\"http://schema.mathworks.com/mf0/Connector/R2020b\"],\"version\":\"1.0\"}"
      mask Display: image('$imagefile'); % Use "Edit Image" on toolstrip to change.
  MOTOR1 : Subsystem
      settings: PortSchema="{\"entries\":[{\"content\":{\"sides\":[{\"content\":{\"connectorIds\":[\"LConn1\",\"LConn2\"]},\"type\":\"ConnectorPlacement.EquallySpacedRectSide\",\"uuid\":\"2895f6cb-f09c-4811-a438-7c51f6a6223f\"},{\"content\":{\"connectorIds\":[\"RConn1\"],\"side\":\"RIGHT\"},\"type\":\"ConnectorPlacement.EquallySpacedRectSide\",\"uuid\":\"62dfe04d-e035-47c8-a996-d867f35d8ae8\"},{\"content\":{\"connectorIds\":[\"LConn3\"],\"side\":\"TOP\"},\"type\":\"ConnectorPlacement.EquallySpacedRectSide\",\"uuid\":\"0c3302b4-833a-415e-90fd-2f2c79a3935c\"}]},\"type\":\"ConnectorPlacement.EquallySpacedConnector\",\"uuid\":\"ac0404f8-73ea-47f6-91f8-dc1d39a3ba60\"}],\"packageUris\":[\"http://schema.mathworks.com/mf0/Connector/R2020b\"],\"version\":\"1.0\"}"
      mask Display: image('$imagefile'); % Use "Edit Image" on toolstrip to change.
  PS-Simulink Converter2 : nesl_utility/PS-Simulink Converter  PhysicalDomain=network_engine_domain  SubClassName=ps_output  LeftPortType=input  RightPortType=output  PseudoPeriodic=off  Frequencies=[]  VectorFormat=inherit  Unit=inherit  AffineConversion=off
  Scope4 : Scope
  Transmission Gear1 : Subsystem
      mask Display: image('$imagefile'); % Use "Edit Image" on toolstrip to change.
  Vehicle chassis1 : Subsystem
      settings: PortSchema="{\"entries\":[{\"content\":{\"sides\":[{\"content\":{\"connectorIds\":[\"LConn1\"]},\"type\":\"ConnectorPlacement.EquallySpacedRectSide\",\"uuid\":\"cbb2d22d-924c-423d-830f-e93cab1699a7\"},{\"content\":{\"side\":\"RIGHT\"},\"type\":\"ConnectorPlacement.EquallySpacedRectSide\",\"uuid\":\"50d26a31-cf69-4945-8446-5696a2ab25a5\"},{\"content\":{\"connectorIds\":[\"LConn2\"],\"side\":\"TOP\"},\"type\":\"ConnectorPlacement.EquallySpacedRectSide\",\"uuid\":\"4303cca7-e79c-4b33-9500-6ba7c742b47b\"}]},\"type\":\"ConnectorPlacement.EquallySpacedConnector\",\"uuid\":\"a196d690-580d-41dc-a9f1-902992004778\"}],\"packageUris\":[\"http://schema.mathworks.com/mf0/Connector/R2020b\"],\"version\":\"1.0\"}"
      mask Display: image('$imagefile'); % Use "Edit Image" on toolstrip to change.
  Conn1 : PMIOPort  Side=Left
  wires:
  PS-Simulink Converter2/1 -> Scope4/1
  connections:
  MOTOR1/RConn1 -- Transmission Gear1/LConn1
  Transmission Gear1/RConn1 -- Vehicle chassis1/LConn1
  Conn1/RConn1 -- MOTOR1/LConn3
  PS-Simulink Converter2/LConn1 -- Vehicle chassis1/LConn2
  Battery1/LConn2 -- MOTOR1/LConn2
  Battery1/LConn1 -- MOTOR1/LConn1

== system PMSM_gm_can_outside_Trq_attack/Transmission Gear ==
  Gear Box : fl_lib/Mechanical/Mechanisms/Gear Box  Tag=varswap  ratio=Gear_ratio  t_in_specify=off  t_in_priority=None  t_in=0 N*m  t_in_nominal_specify=off  t_in_nominal_unit=N*m  t_in_nominal_value=1  t_out_specify=off  t_out_priority=None  t_out=0 N*m  t_out_nominal_specify=off  t_out_nominal_unit=N*m  t_out_nominal_value=1
  Ideal Torque Sensor : fl_lib/Mechanical/Mechanical Sensors/Ideal Torque Sensor
  PS-Simulink Converter1 : nesl_utility/PS-Simulink Converter  PhysicalDomain=network_engine_domain  SubClassName=ps_output  LeftPortType=input  RightPortType=output  PseudoPeriodic=off  Frequencies=[]  VectorFormat=inherit  Unit=inherit  AffineConversion=off
  To Workspace1 : ToWorkspace  VariableName=T_measured  SaveFormat=Timeseries  SampleTime=-1
  Connection Port1 : PMIOPort  Side=Right
  Connection Port : PMIOPort  Port=2  Side=Left
  tag scope: T_meas=global
  wires:
  PS-Simulink Converter1/1 -> To Workspace1/1, [T_meas]  "T_meas"
  connections:
  Ideal Torque Sensor/RConn1 -- Gear Box/LConn1
  Connection Port1/RConn1 -- Gear Box/RConn1
  Connection Port/RConn1 -- Ideal Torque Sensor/LConn1
  PS-Simulink Converter1/LConn1 -- Ideal Torque Sensor/RConn2

== system PMSM_gm_can_outside_Trq_attack/Triggered Subsystem ==
  Input : Inport
  Trigger : TriggerPort  TriggerType=function-call  VariantControl=(inherit)
  CAN Unpack : canmsglib/CAN Unpack  CANdbFile=C:\Users\Sadek\OneDrive - Politecnico di Torino\Final model\can_ecu.dbc  MsgList=Velocity_Reference  MsgName=Velocity_Reference  MsgIDType=Standard (11-bit identifier)  MsgIdentifier=2  MsgLength=8  SignalInfo={'Velocity_Reference_Signal','0','64','LE','double','Standard','0','1','-20','0','10000'}  IDPort=off  TimestampPort=off  ErrorPort=off  RemotePort=off  LengthPort=off  StatusPort=off  ApplyMinMax=off
      settings: LibrarySourceBlock=canlib/CAN Unpack  DataFormat=CANdb specified signals
  V_ref : Outport
  wires:
  Input/1 -> CAN Unpack/1
  CAN Unpack/1 -> V_ref/1

== system PMSM_gm_can_outside_Trq_attack/Triggered Subsystem1 ==
  Input : Inport
  Trigger : TriggerPort  TriggerType=function-call  VariantControl=(inherit)
  CAN Unpack : canmsglib/CAN Unpack  CANdbFile=C:\Users\Sadek\OneDrive - Politecnico di Torino\Final model\can_ecu.dbc  MsgList=Velocity_Feedback  MsgName=Velocity_Feedback  MsgIDType=Standard (11-bit identifier)  MsgIdentifier=1  MsgLength=8  SignalInfo={'Velocity_Feedback_Signal','0','64','LE','double','Standard','0','1','-20','0','10000'}  IDPort=off  TimestampPort=off  ErrorPort=off  RemotePort=off  LengthPort=off  StatusPort=off  ApplyMinMax=off
      settings: LibrarySourceBlock=canlib/CAN Unpack  DataFormat=CANdb specified signals
  V_fdbk : Outport
  wires:
  Input/1 -> CAN Unpack/1
  CAN Unpack/1 -> V_fdbk/1

== system PMSM_gm_can_outside_Trq_attack/Triggered Subsystem2 ==
  Input : Inport
  Trigger : TriggerPort  TriggerType=function-call  VariantControl=Variant
  CAN Unpack : canmsglib/CAN Unpack  CANdbFile=C:\Users\Sadek\OneDrive - Politecnico di Torino\Final model\can_ecu.dbc  MsgList=Motor_Torque  MsgName=Motor_Torque  MsgIDType=Standard (11-bit identifier)  MsgIdentifier=0  MsgLength=8  SignalInfo={'Motor_Torque_Signal','0','64','LE','signed','Standard','0','1','-20','-50000','50000'}  IDPort=off  TimestampPort=off  ErrorPort=off  RemotePort=off  LengthPort=off  StatusPort=off  ApplyMinMax=off
      settings: LibrarySourceBlock=canlib/CAN Unpack  DataFormat=CANdb specified signals
  Outport : Outport
  wires:
  Input/1 -> CAN Unpack/1
  CAN Unpack/1 -> Outport/1

== system PMSM_gm_can_outside_Trq_attack/Triggered Subsystem3 ==
  Input : Inport
  Trigger : TriggerPort  TriggerType=function-call  VariantControl=Variant
  CAN Unpack : canmsglib/CAN Unpack  CANdbFile=C:\Users\Sadek\OneDrive - Politecnico di Torino\Final model\can_ecu.dbc  MsgList=SOC  MsgName=SOC  MsgIDType=Standard (11-bit identifier)  MsgIdentifier=5  MsgLength=8  SignalInfo={'SOC_signal','0','64','LE','double','Standard','0','1','-20','0','100'}  IDPort=off  TimestampPort=off  ErrorPort=off  RemotePort=off  LengthPort=off  StatusPort=off  ApplyMinMax=off
      settings: LibrarySourceBlock=canlib/CAN Unpack  DataFormat=CANdb specified signals
  Gain : Gain  Gain=100
  Outport : Outport
  wires:
  CAN Unpack/1 -> Gain/1
  Input/1 -> CAN Unpack/1
  Gain/1 -> Outport/1

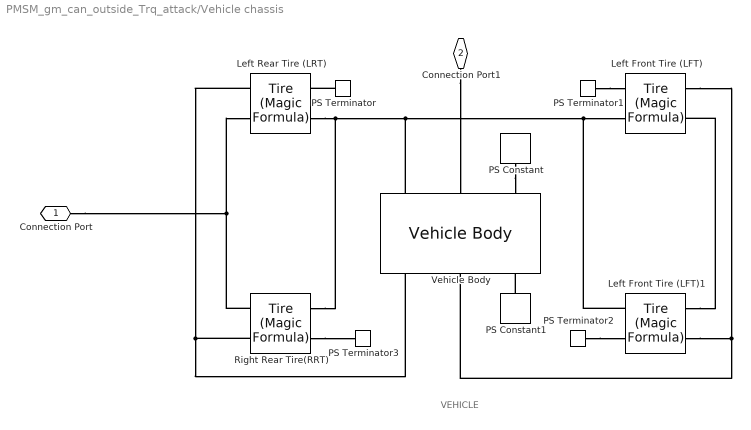
== system PMSM_gm_can_outside_Trq_attack/Vehicle chassis ==
  note: VEHICLE
  Left Front Tire (LFT) : sdl_lib/Tires & Vehicles/Tire (Magic Formula)  parameterization=sdl.enum.magic_tire_model.load  F_z1=3000 N  F_x1=3500 N  kappa1=10  B_m=10  C_m=1.9  D_m=1  E_m=0.97  fz0=3500 N  p_Cx=1.685  p_Dx=[1.21, -.037]  p_Ex=[.344, .095, -.02, 0]  p_Kx=[21.51, -.163, .245]  p_Hx=[-.002, .002]  p_Vx=[0, 0]  rolling_radius_model=sdl.enum.RollingRadiusParameterization.Constant  r_e=Tire_rad m  r_0=0.3 m  breff=8.39  dreff=0.26  freff=0.074  q_re0=0.99  q_v1=0.008  longvl=17 m/s  cz=5e5 N/m  model_resistance=true  resistance_model=sdl.enum.rollingResistanceParameterization.constant  coeff=0.022  p_tire=250e3 Pa  alpha=-0.003  beta=0.97  coeff_a=84e-4  coeff_b=6.2e-4 s/m  coeff_c=1.6e-4 s^2/m^2  p_tire0=240e3 Pa  fz0_resistance=4000 N  vH0=16 m/s  q_Sy=[.0082, 0, .0014, .001, 0, 0, 1.08, -.5]  v_thr=0.001 m/s  enable_scaling_coefficients=false  lfzO=1  lcx=1  lmux=1  lex=1  lkx=1  lhx=1  lvx=1  lmy=1  model_compliance=sdl.enum.compliance.off  stiffness=1e6 N/m  damping=1000 N*s/m  model_inertia=sdl.enum.model_inertia.on  inertia=1 kg*m^2  initial_velocity=0 rad/s  vxlow=1 m/s  v_tr_thr=0.1 m/s  kpumin=-1.5  kpumax=1.5
  Left Front Tire (LFT)1 : sdl_lib/Tires & Vehicles/Tire (Magic Formula)  parameterization=sdl.enum.magic_tire_model.load  F_z1=3000 N  F_x1=3500 N  kappa1=10  B_m=10  C_m=1.9  D_m=1  E_m=0.97  fz0=3500 N  p_Cx=1.685  p_Dx=[1.21, -.037]  p_Ex=[.344, .095, -.02, 0]  p_Kx=[21.51, -.163, .245]  p_Hx=[-.002, .002]  p_Vx=[0, 0]  rolling_radius_model=sdl.enum.RollingRadiusParameterization.Constant  r_e=Tire_rad m  r_0=0.3 m  breff=8.39  dreff=0.26  freff=0.074  q_re0=0.99  q_v1=0.008  longvl=17 m/s  cz=5e5 N/m  model_resistance=true  resistance_model=sdl.enum.rollingResistanceParameterization.constant  coeff=0.022  p_tire=250e3 Pa  alpha=-0.003  beta=0.97  coeff_a=84e-4  coeff_b=6.2e-4 s/m  coeff_c=1.6e-4 s^2/m^2  p_tire0=240e3 Pa  fz0_resistance=4000 N  vH0=16 m/s  q_Sy=[.0082, 0, .0014, .001, 0, 0, 1.08, -.5]  v_thr=0.001 m/s  enable_scaling_coefficients=false  lfzO=1  lcx=1  lmux=1  lex=1  lkx=1  lhx=1  lvx=1  lmy=1  model_compliance=sdl.enum.compliance.off  stiffness=1e6 N/m  damping=1000 N*s/m  model_inertia=sdl.enum.model_inertia.on  inertia=1 kg*m^2  initial_velocity=0 rad/s  vxlow=1 m/s  v_tr_thr=0.1 m/s  kpumin=-1.5  kpumax=1.5
  Left Rear Tire (LRT) : sdl_lib/Tires & Vehicles/Tire (Magic Formula)  parameterization=sdl.enum.magic_tire_model.load  F_z1=3000 N  F_x1=3500 N  kappa1=10  B_m=10  C_m=1.9  D_m=1  E_m=0.97  fz0=3500 N  p_Cx=1.685  p_Dx=[1.21, -.037]  p_Ex=[.344, .095, -.02, 0]  p_Kx=[21.51, -.163, .245]  p_Hx=[-.002, .002]  p_Vx=[0, 0]  rolling_radius_model=sdl.enum.RollingRadiusParameterization.Constant  r_e=Tire_rad m  r_0=0.3 m  breff=8.39  dreff=0.26  freff=0.074  q_re0=0.99  q_v1=0.008  longvl=17 m/s  cz=5e5 N/m  model_resistance=true  resistance_model=sdl.enum.rollingResistanceParameterization.constant  coeff=0.022  p_tire=250e3 Pa  alpha=-0.003  beta=0.97  coeff_a=84e-4  coeff_b=6.2e-4 s/m  coeff_c=1.6e-4 s^2/m^2  p_tire0=240e3 Pa  fz0_resistance=4000 N  vH0=16 m/s  q_Sy=[.0082, 0, .0014, .001, 0, 0, 1.08, -.5]  v_thr=0.001 m/s  enable_scaling_coefficients=false  lfzO=1  lcx=1  lmux=1  lex=1  lkx=1  lhx=1  lvx=1  lmy=1  model_compliance=sdl.enum.compliance.off  stiffness=1e6 N/m  damping=1000 N*s/m  model_inertia=sdl.enum.model_inertia.on  inertia=1 kg*m^2  initial_velocity=0 rad/s  vxlow=1 m/s  v_tr_thr=0.1 m/s  kpumin=-1.5  kpumax=1.5
  PS Constant : fl_lib/Physical Signals/Sources/PS Constant  constant=0 m/s
  PS Constant1 : fl_lib/Physical Signals/Sources/PS Constant  constant=0 deg
  PS Terminator{,1..3} (4 alike) : fl_lib/Physical Signals/Sinks/PS Terminator
  Right Rear Tire(RRT) : sdl_lib/Tires & Vehicles/Tire (Magic Formula)  parameterization=sdl.enum.magic_tire_model.load  F_z1=3000 N  F_x1=3500 N  kappa1=10  B_m=10  C_m=1.9  D_m=1  E_m=0.97  fz0=3500 N  p_Cx=1.685  p_Dx=[1.21, -.037]  p_Ex=[.344, .095, -.02, 0]  p_Kx=[21.51, -.163, .245]  p_Hx=[-.002, .002]  p_Vx=[0, 0]  rolling_radius_model=sdl.enum.RollingRadiusParameterization.Constant  r_e=Tire_rad m  r_0=0.3 m  breff=8.39  dreff=0.26  freff=0.074  q_re0=0.99  q_v1=0.008  longvl=17 m/s  cz=5e5 N/m  model_resistance=true  resistance_model=sdl.enum.rollingResistanceParameterization.constant  coeff=0.022  p_tire=250e3 Pa  alpha=-0.003  beta=0.97  coeff_a=84e-4  coeff_b=6.2e-4 s/m  coeff_c=1.6e-4 s^2/m^2  p_tire0=240e3 Pa  fz0_resistance=4000 N  vH0=16 m/s  q_Sy=[.0082, 0, .0014, .001, 0, 0, 1.08, -.5]  v_thr=0.001 m/s  enable_scaling_coefficients=false  lfzO=1  lcx=1  lmux=1  lex=1  lkx=1  lhx=1  lvx=1  lmy=1  model_compliance=sdl.enum.compliance.off  stiffness=1e6 N/m  damping=1000 N*s/m  model_inertia=sdl.enum.model_inertia.on  inertia=1 kg*m^2  initial_velocity=0 rad/s  vxlow=1 m/s  v_tr_thr=0.1 m/s  kpumin=-1.5  kpumax=1.5
  Vehicle Body : sdl_lib/Tires & Vehicles/Vehicle Body  mass=mass kg  n_w=2  x_f=1.4 m  x_r=1.6 m  y_c=0.5 m  mass_var=simscape.enum.onoff.off  g=9.81 m/s^2  liftoff_warning=simscape.enum.onoff.off  area=fr_area m^2  Cd=drag_coeff  rho=1.225 kg/m^3  model_pitch=simscape.enum.onoff.off  inertia=4000 kg*m^2  suspension_model=sdl.enum.linearTLU.linear  k_f=1e4 N/m  b_f=1e4 N*s/m  k_r=1e4 N/m  b_r=1e4 N*s/m  k_f_TLU=[-2000, -1000, 0, 1000, 2000] N  x_f_TLU=[-.4, -.2, 0, .2, .4] m  b_f_TLU=[-200, -100, 0, 100, 200] N  v_f_TLU=[-4, -2, 0, 2, 4] m/s  k_r_TLU=[-2000, -1000, 0, 1000, 2000] N  x_r_TLU=[-.4, -.2, 0, .2, .4] m  b_r_TLU=[-200, -100, 0, 100, 200] N  v_r_TLU=[-4, -2, 0, 2, 4] m/s  interp_method=simscape.enum.interpolation.linear  extrap_method=simscape.enum.extrapolation.linear  model_hardstop=simscape.enum.onoff.off  upper_bound_f=.25 m  lower_bound_f=-.25 m  stop_k_f=1e6 N/m  stop_b_f=150 N*s/m  upper_bound_r=.25 m  lower_bound_r=-.25 m  stop_k_r=1e6 N/m  stop_b_r=150 N*s/m  initial_pitch=0 rad  initial_pitch_rate=0 rad/s  v_specify=off  v_priority=High  v=0 m/s  v_nominal_specify=off  v_nominal_unit=m/s  v_nominal_value=1
  Connection Port : PMIOPort  Side=Left
  Connection Port1 : PMIOPort  Port=2  Side=Left
  connections:
  Right Rear Tire(RRT)/LConn2 -- Connection Port/RConn1 -- Left Rear Tire (LRT)/LConn2
  Left Front Tire (LFT)1/LConn1 -- Vehicle Body/RConn2 -- Left Front Tire (LFT)/LConn1
  Right Rear Tire(RRT)/RConn2 -- Left Rear Tire (LRT)/RConn2 -- Vehicle Body/LConn1 -- Left Front Tire (LFT)1/RConn2 -- Left Front Tire (LFT)/RConn2
  Vehicle Body/RConn1 -- Left Rear Tire (LRT)/LConn1 -- Right Rear Tire(RRT)/LConn1
  PS Terminator1/LConn1 -- Left Front Tire (LFT)/RConn1
  PS Terminator/LConn1 -- Left Rear Tire (LRT)/RConn1
  PS Terminator2/LConn1 -- Left Front Tire (LFT)1/RConn1
  PS Constant/RConn1 -- Vehicle Body/LConn3
  Left Front Tire (LFT)1/LConn2 -- Left Front Tire (LFT)/LConn2
  Connection Port1/RConn1 -- Vehicle Body/LConn2
  PS Constant1/RConn1 -- Vehicle Body/RConn3
  Right Rear Tire(RRT)/RConn1 -- PS Terminator3/LConn1

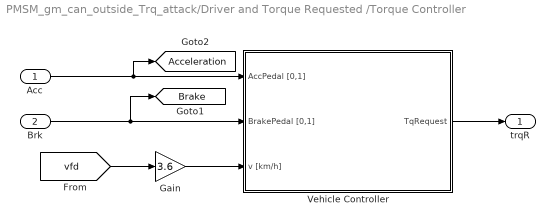
== system PMSM_gm_can_outside_Trq_attack/Driver and Torque Requested /Torque Controller ==
  Acc : Inport
  Brk : Inport  Port=2
  Gain : Gain  Gain=3.6
  Vehicle Controller : Subsystem
  trqR : Outport  VectorParamsAs1DForOutWhenUnconnected=off
  tag scope: Acceleration=global, Brake=global
  wires:
  Vehicle Controller/1(TqRequest) -> trqR/1
  Acc/1 -> Vehicle Controller/1(AccPedal [0,1]), [Acceleration]
  Brk/1 -> [Brake], Vehicle Controller/2(BrakePedal [0,1])
  [vfd] -> Gain/1
  Gain/1 -> Vehicle Controller/3(v [km/h])

== system PMSM_gm_can_outside_Trq_attack/SOC calculation /SOC calculation ==
  I [A] : Inport
  1/(nominal battery capacity) : Gain  Gain=1/(Rated_Cap*3600)
  Discrete-Time Integrator : DiscreteIntegrator  SampleTime=-1  ICPrevOutput=DiscIntNeverNeededParam  ICPrevScaledInput=DiscIntNeverNeededParam
  Initial SOC : Constant  Value=SOC0
  Rate Transition2 : RateTransition
  Sum2 : Sum  Inputs=+-
  SOC [0,1] : Outport  VectorParamsAs1DForOutWhenUnconnected=off
  wires:
  I [A]/1 -> Rate Transition2/1
  Rate Transition2/1 -> 1/(nominal battery capacity)/1
  1/(nominal battery capacity)/1 -> Discrete-Time Integrator/1
  Initial SOC/1 -> Sum2/1
  Discrete-Time Integrator/1 -> Sum2/2
  Sum2/1 -> SOC [0,1]/1

== system PMSM_gm_can_outside_Trq_attack/SOC calculation /Sensing current ==
  Current Sensor : fl_lib/Electrical/Electrical Sensors/Current Sensor
  PS-Simulink Converter2 : nesl_utility/PS-Simulink Converter  PhysicalDomain=network_engine_domain  SubClassName=ps_output  LeftPortType=input  RightPortType=output  PseudoPeriodic=off  Frequencies=[]  VectorFormat=1-D array  Unit=A  AffineConversion=off
  + : PMIOPort  Side=Left
  - : PMIOPort  Port=2  Side=Right
  Out1 : Outport  VectorParamsAs1DForOutWhenUnconnected=off
  wires:
  PS-Simulink Converter2/1 -> Out1/1
  connections:
  -/RConn1 -- Current Sensor/RConn2
  Current Sensor/RConn1 -- PS-Simulink Converter2/LConn1
  Current Sensor/LConn1 -- +/RConn1
